simulink model "lab4_task1"  (R2020a)
settings: Solver=FixedStepAuto  StartTime=0.0  StopTime=inf  RelTol=1e-3
model workspace (MAT data in the model file):
  SL_ROS_VariableLengthArrays_MaxSizes.CommonInfo.ArrayTruncateAction = 'EmitWarning'
  SL_ROS_VariableLengthArrays_MaxSizes.MsgTypeMap = containers.Map
  SL_ROS_VariableLengthArrays_MaxSizes.MsgTypeMap.serialization.keys = {'sensor_msgs/LaserScan'}
  SL_ROS_VariableLengthArrays_MaxSizes.MsgTypeMap.serialization.values{1}(1).PropertyName = 'Intensities'
  SL_ROS_VariableLengthArrays_MaxSizes.MsgTypeMap.serialization.values{1}(1).DataType = 'single'
  SL_ROS_VariableLengthArrays_MaxSizes.MsgTypeMap.serialization.values{1}(1).MaxLength = 360
  SL_ROS_VariableLengthArrays_MaxSizes.MsgTypeMap.serialization.values{1}(2).PropertyName = 'Ranges'
  SL_ROS_VariableLengthArrays_MaxSizes.MsgTypeMap.serialization.values{1}(2).DataType = 'single'
  SL_ROS_VariableLengthArrays_MaxSizes.MsgTypeMap.serialization.values{1}(2).MaxLength = 360
  SL_ROS_VariableLengthArrays_MaxSizes.MsgTypeMap.serialization.uniformity = 0
  SL_ROS_VariableLengthArrays_MaxSizes.MsgTypeMap.serialization.keyType = 'char'
  SL_ROS_VariableLengthArrays_MaxSizes.MsgTypeMap.serialization.valueType = 'any'
values from neighbouring files (symbols this model uses):
  theta = ang + curr_yaw    [live_repulsion.m]
undefined symbols (not defined in the file or in its folder): angdiff, Angular, Linear, X, Y
libraries: simulink x9, robotlib x4, robotcorelib x1, simulink_extras x1
settings Model: Creator=Sina  LastModifiedBy=Pablo
settings DataIOCC: ReturnWorkspaceOutputs=off
settings OptimizationCC: EnhancedBackFolding=on  PassReuseOutputArgsAs=Individual arguments  ZeroExternalMemoryAtStartup=off  ZeroInternalMemoryAtStartup=off  MaxStackSize=64  OptimizeBlockOrder=speed  DifferentSizesBufferReuse=on  OptimizationCustomize=off  EfficientTunableParamExpr=on
settings DebuggingCC: ParameterTunabilityLossMsg=error  ArithmeticOperatorsInVariantConditions=warning
settings HardwareCC: ProdBitPerPointer=32  ProdBitPerSizeT=32  ProdBitPerPtrDiffT=32  ProdLargestAtomicFloat=None  ProdIntDivRoundTo=Undefined  ProdEndianess=Unspecified  ProdWordSize=32  ProdHWDeviceType=Generic->Unspecified (assume 32-bit Generic)  UseEmbeddedCoderFeatures=off
settings SFSimCC: SimUseLocalCustomCode=off  MATLABDynamicMemAlloc=off  CustomCodeUndefinedFunction=UseInterfaceOnly
settings RTWCC: SystemTargetFile=ert.tlc  HardwareBoard=Robot Operating System (ROS)  TemplateMakefile=ert_default_tmf  RTWUseLocalCustomCode=off  Toolchain=Catkin  TargetLang=C++
settings CodeAppCC: ForceParamTrailComments=on  IgnoreCustomStorageClasses=off  OperatorAnnotations=on  SimulinkDataObjDesc=on  SFDataObjDesc=on  InsertBlockDesc=on
settings ERTTargetCC: SupportNonInlinedSFcns=on

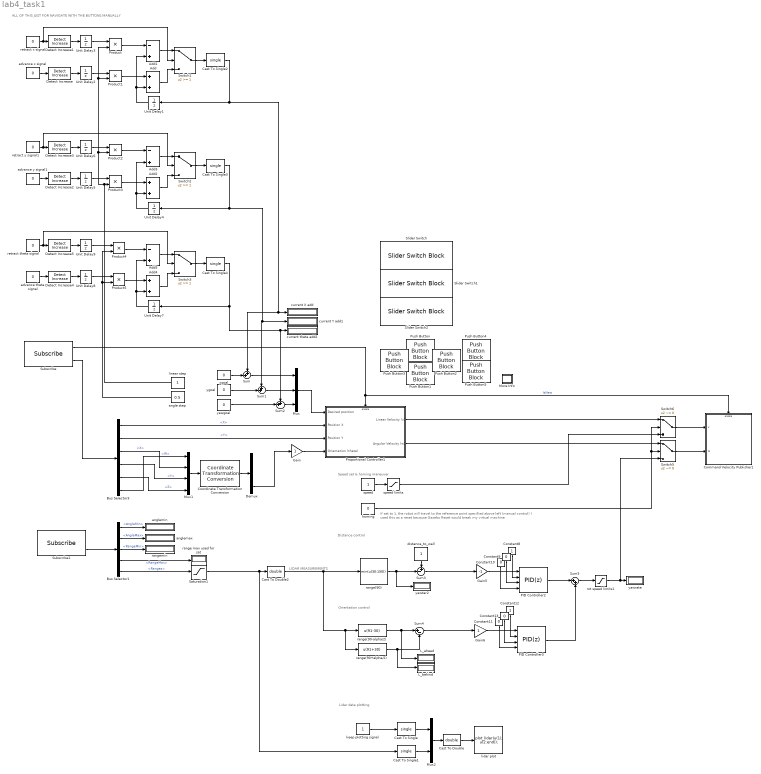
== system lab4_task1 ==
  note: ALL OF THIS JUST FOR NAVIGATE WITH THE BUTTONS MANUALLY
  note: LIDAR MEASUREMENTS
  note: if set to 1, the robot will travel to the reference point specified above left (manual control)
      | I used this as a reset because Gazebo Reset would break my virtual machine
  note: Speed set & homing maneuver
  note: Orientation control
  note: Distance control
  note: Lidar data plotting
  Add : Sum
  Add1 : Sum  Inputs=-+
  Add2 : Sum
  Add3 : Sum  Inputs=-+
  Add4 : Sum
  Add5 : Sum  Inputs=-+
  Bus Selector1 : BusSelector  OutputSignals=AngleMin,AngleMax,RangeMin,RangeMax,Ranges
  Bus Selector3 : BusSelector  OutputSignals=Pose.Pose.Position.X,Pose.Pose.Position.Y,Pose.Pose.Orientation.X,Pose.Pose.Orientation.Y,Pose.Pose.Orientation.Z,Pose.Pose.Orientation.W
  Cast To Double : DataTypeConversion  OutDataTypeStr=double
  Cast To Double2 : DataTypeConversion  OutDataTypeStr=double
  Cast To Single{,1..4} (5 alike) : DataTypeConversion  OutDataTypeStr=single
  Command Velocity Publisher1 : Subsystem
  Constant{9..11,13} (4 alike) : Constant  Value=0
  Constant12 : Constant
  Constant8 : Constant
  Coordinate Transformation Conversion : robotcorelib/Coordinate Transformation Conversion  InputRepresentation=Quaternion  InputEulerSequence=XYZ  ShowTrVecInputPort=on  OutputRepresentation=Euler Angles  OutputEulerSequence=XYZ  ShowTrVecOutputPort=on  SimulateUsing=Interpreted execution
      settings: SourceProductBaseCode=NV,RO,RR
  Demux : Demux  Outputs=3
  Detect Increase{,1..5} (6 alike) : simulink/Logic and Bit Operations/Detect Increase  vinit=0.0  OutDataTypeStr=boolean
  Gain : Gain
  Gain5 : Gain  Gain=-1
  Gain6 : Gain
  L_ahead : Display
  L_behind : Display
  More Info : Subsystem
      settings: OpenFcn=showdemo(bdroot(gcb))
      mask Display: disp('?')
  Mux : Mux  Inputs=3
  Mux1 : Mux
  Mux2 : Mux  Inputs=2
  PID Controller2 : simulink/Continuous/PID Controller  Controller=PID  Form=Parallel  TimeDomain=Discrete-time  UseExternalTs=off  SampleTime=-1  IntegratorMethod=Forward Euler  FilterMethod=Forward Euler  ControllerParametersSource=external  P=1  I=1  D=0  UseFilter=off  N=100  TunerSelectOption=Transfer Function Based (PID Tuner App)  InitialConditionSource=internal  InitialConditionForIntegrator=0  InitialConditionForFilter=0  DifferentiatorICPrevScaledInput=0  ExternalReset=none  TrackingMode=off  Kt=1  LimitOutput=off  UpperSaturationLimit=inf  LowerSaturationLimit=-inf  LinearizeAsGain=on  AntiWindupMode=none  Kb=1  POutMin=[]  POutMax=[]  IOutMin=[]  IOutMax=[]  DOutMin=[]  DOutMax=[]  NOutMin=[]  NOutMax=[]  SumOutMin=[]  SumOutMax=[]  SaturationOutMin=[]  SaturationOutMax=[]  PParamMin=[]  PParamMax=[]  IParamMin=[]  IParamMax=[]  DParamMin=[]  DParamMax=[]  NParamMin=[]  NParamMax=[]  KbParamMin=[]  KbParamMax=[]  KtParamMin=[]  KtParamMax=[]  KbOutMin=[]  KbOutMax=[]  KtOutMin=[]  KtOutMax=[]  IntegratorOutMin=[]  IntegratorOutMax=[]  FilterOutMin=[]  FilterOutMax=[]  SumI1OutMin=[]  SumI1OutMax=[]  SumI2OutMin=[]  SumI2OutMax=[]  SumI3OutMin=[]  SumI3OutMax=[]  SumI4OutMin=[]  SumI4OutMax=[]  SumDOutMin=[]  SumDOutMax=[]  DifferentiatorOutMin=[]  DifferentiatorOutMax=[]  FilterDiffOutCoefMin=[]  FilterDiffOutCoefMax=[]  ReciprocalOutMin=[]  ReciprocalOutMax=[]  SumDenOutMin=[]  SumDenOutMax=[]  SumNumOutMin=[]  SumNumOutMax=[]  DivideOutMin=[]  DivideOutMax=[]  UdiffTsProdOutMin=[]  UdiffTsProdOutMax=[]  NTsProdOutMin=[]  NTsProdOutMax=[]  UintegralTsProdOutMin=[]  UintegralTsProdOutMax=[]  UngainTsProdOutMin=[]  UngainTsProdOutMax=[]  IntegratorContinuousStateAttributes=''  IntegratorStateMustResolveToSignalObject=off  IntegratorRTWStateStorageClass=Auto  FilterContinuousStateAttributes=''  FilterStateMustResolveToSignalObject=off  FilterRTWStateStorageClass=Auto  ParallelPVariant=ExternalParameters  IdealPVariant=Disabled  IVariant=ExternalParameters  DVariant=ExternalParameters  IntegratorVariant=Discrete  SatVariant=Disabled  AWVariant=Passthrough  PCopyVariant=Disabled  TRVariant=Disabled  FdbkBlocksVariant=Forward  IdealPFdbkVariant=Disabled  SatFdbkVariant=Disabled  DerivativeFilterVariant=Differentiator  NVariant=Passthrough  NCopyVariant=Disabled_SignalSpec  FilterICVariant=InternalICsDifferentiator  IntegratorICVariant=InternalICs  ExternalResetVariant=Disabled  TRSumVariant=Passthrough  SumFdbkVariant=Disabled  SumVariant=Sum_PID  TsampFilterVariant=InternalTs  TsampNgainVariant=Passthrough  TsampIntegralVariant=Passthrough
  PID Controller3 : simulink/Continuous/PID Controller  Controller=PID  Form=Parallel  TimeDomain=Discrete-time  UseExternalTs=off  SampleTime=-1  IntegratorMethod=Forward Euler  FilterMethod=Forward Euler  ControllerParametersSource=external  P=1  I=1  D=0  UseFilter=off  N=100  TunerSelectOption=Transfer Function Based (PID Tuner App)  InitialConditionSource=internal  InitialConditionForIntegrator=0  InitialConditionForFilter=0  DifferentiatorICPrevScaledInput=0  ExternalReset=none  TrackingMode=off  Kt=1  LimitOutput=off  UpperSaturationLimit=inf  LowerSaturationLimit=-inf  LinearizeAsGain=on  AntiWindupMode=none  Kb=1  POutMin=[]  POutMax=[]  IOutMin=[]  IOutMax=[]  DOutMin=[]  DOutMax=[]  NOutMin=[]  NOutMax=[]  SumOutMin=[]  SumOutMax=[]  SaturationOutMin=[]  SaturationOutMax=[]  PParamMin=[]  PParamMax=[]  IParamMin=[]  IParamMax=[]  DParamMin=[]  DParamMax=[]  NParamMin=[]  NParamMax=[]  KbParamMin=[]  KbParamMax=[]  KtParamMin=[]  KtParamMax=[]  KbOutMin=[]  KbOutMax=[]  KtOutMin=[]  KtOutMax=[]  IntegratorOutMin=[]  IntegratorOutMax=[]  FilterOutMin=[]  FilterOutMax=[]  SumI1OutMin=[]  SumI1OutMax=[]  SumI2OutMin=[]  SumI2OutMax=[]  SumI3OutMin=[]  SumI3OutMax=[]  SumI4OutMin=[]  SumI4OutMax=[]  SumDOutMin=[]  SumDOutMax=[]  DifferentiatorOutMin=[]  DifferentiatorOutMax=[]  FilterDiffOutCoefMin=[]  FilterDiffOutCoefMax=[]  ReciprocalOutMin=[]  ReciprocalOutMax=[]  SumDenOutMin=[]  SumDenOutMax=[]  SumNumOutMin=[]  SumNumOutMax=[]  DivideOutMin=[]  DivideOutMax=[]  UdiffTsProdOutMin=[]  UdiffTsProdOutMax=[]  NTsProdOutMin=[]  NTsProdOutMax=[]  UintegralTsProdOutMin=[]  UintegralTsProdOutMax=[]  UngainTsProdOutMin=[]  UngainTsProdOutMax=[]  IntegratorContinuousStateAttributes=''  IntegratorStateMustResolveToSignalObject=off  IntegratorRTWStateStorageClass=Auto  FilterContinuousStateAttributes=''  FilterStateMustResolveToSignalObject=off  FilterRTWStateStorageClass=Auto  ParallelPVariant=ExternalParameters  IdealPVariant=Disabled  IVariant=ExternalParameters  DVariant=ExternalParameters  IntegratorVariant=Discrete  SatVariant=Disabled  AWVariant=Passthrough  PCopyVariant=Disabled  TRVariant=Disabled  FdbkBlocksVariant=Forward  IdealPFdbkVariant=Disabled  SatFdbkVariant=Disabled  DerivativeFilterVariant=Differentiator  NVariant=Passthrough  NCopyVariant=Disabled_SignalSpec  FilterICVariant=InternalICsDifferentiator  IntegratorICVariant=InternalICs  ExternalResetVariant=Disabled  TRSumVariant=Passthrough  SumFdbkVariant=Disabled  SumVariant=Sum_PID  TsampFilterVariant=InternalTs  TsampNgainVariant=Passthrough  TsampIntegralVariant=Passthrough
  Product{,1..5} (6 alike) : Product
  Proportional Controller1 : Subsystem
  Push Button : PushButtonBlock  ButtonText=X+
  Push Button1 : PushButtonBlock  ButtonText=X-
  Push Button2 : PushButtonBlock  ButtonText=Y+
  Push Button3 : PushButtonBlock  ButtonText=Y-
  Push Button4 : PushButtonBlock  ButtonText=theta+
  Push Button5 : PushButtonBlock  ButtonText=theta-
  Saturation1 : Saturate  UpperLimit=3.6  LowerLimit=-20  LinearizeAsGain=off
  Slider Switch : SliderSwitchBlock
      settings: Values={{'STOP OFF', 'STOP ON'}, [0 1]}
  Slider Switch1 : SliderSwitchBlock
      settings: Values={{'PLOT OFF', 'PLOT ON'}, [0 1]}
  Slider Switch2 : SliderSwitchBlock
      settings: Values={{'YAW OFF', 'YAW ON'}, [0 -1]}
  Subscribe : robotlib/Subscribe  topicSource=Select from ROS network  topic=/odom  messageType=nav_msgs/Odometry  sampleTime=-1  messageQueueLength=51
  Subscribe1 : robotlib/Subscribe  topicSource=Select from ROS network  topic=/scan  messageType=sensor_msgs/LaserScan  sampleTime=-1  messageQueueLength=51
  Sum : Sum  Inputs=++|
  Sum1 : Sum  Inputs=++|
  Sum2 : Sum  Inputs=++|
  Sum3 : Sum  Inputs=+-|
  Sum4 : Sum  Inputs=|+-
  Sum5 : Sum  Inputs=|++
  Switch1 : Switch  Threshold=1
  Switch2 : Switch  Threshold=1
  Switch3 : Switch  Threshold=1
  Switch5 : Switch  Criteria=u2 ~= 0
  Switch6 : Switch  Criteria=u2 ~= 0
  Unit Delay{1..9} (9 alike) : UnitDelay  SampleTime=-1  HasFrameUpgradeWarning=on
  advance theta signal : Constant  Value=0
  advance x signal : Constant  Value=0
  advance y signal1 : Constant  Value=0
  angle step : Constant  Value=0.5
  anglemax : Display
  anglemin : Display
  current X add : Display
  current Y add1 : Display
  current theta add2 : Display
  distance_to_wall : Constant
  homing : Constant  Value=0
  keep plotting signal : Constant
  lidar plot : MATLABFcn  MATLABFcn=plot_lidar(u(1), u(2:end));  OutputDimensions=1  Output1D=off
  linear step : Constant
  range max used for sat : Display
  range(90) : MATLABFcn  MATLABFcn=min(u(30:150))  OutputDimensions=1  Output1D=off
  range(90+alpha/2) : MATLABFcn  MATLABFcn=u(91+30)  OutputDimensions=1  Output1D=off
  range(90-alpha/2) : MATLABFcn  MATLABFcn=u(91-30)  OutputDimensions=1  Output1D=off
  rangemin : Display
  retract theta signal : Constant  Value=0
  retract x signal : Constant  Value=0
  retract y signal1 : Constant  Value=0
  rot speed limits1 : Saturate  LinearizeAsGain=off
  speed : Constant
  speed limits : Saturate  UpperLimit=0.3  LowerLimit=-0.3  LinearizeAsGain=off
  xgoal : Constant  Value=0
  yawgoal : Constant  Value=0
  yawrate : Display
  yawtar2 : Display
  ygoal : Constant  Value=0
  wires:
  Bus Selector3/2 -> Proportional Controller1/3(Position Y)  "<Y>"
  Bus Selector3/1 -> Proportional Controller1/2(Position X)  "<X>"
  Subscribe/1 -> Command Velocity Publisher1/Enable, Proportional Controller1/Enable  "IsNew"
  Bus Selector3/5 -> Mux1/4  "<Z>"
  Bus Selector3/3 -> Mux1/2  "<X>"
  Subscribe/2 -> Bus Selector3/1
  Bus Selector3/4 -> Mux1/3  "<Y>"
  Bus Selector3/6 -> Mux1/1  "<W>"
  Bus Selector1/2 -> anglemax/1  "<AngleMax>"
  Bus Selector1/5 -> Saturation1/1  "<Ranges>"
  Subscribe1/2 -> Bus Selector1/1
  Bus Selector1/1 -> anglemin/1  "<AngleMin>"
  Mux1/1 -> Coordinate Transformation Conversion/1
  Gain/1 -> Proportional Controller1/4(Orientation (theta))
  Mux/1 -> Proportional Controller1/1(Desired position)
  Coordinate Transformation Conversion/1 -> Demux/1
  Demux/3 -> Gain/1
  Bus Selector1/3 -> rangemin/1  "<RangeMin>"
  Bus Selector1/4 -> range max used for sat/1  "<RangeMax>"
  advance x signal/1 -> Detect Increase/1
  Add/1 -> Switch1/3
  Unit Delay1/1 -> Add/2, Add1/2
  retract x signal/1 -> Switch1/2, Detect Increase1/1
  Add1/1 -> Switch1/1
  Detect Increase/1 -> Unit Delay2/1
  Detect Increase1/1 -> Unit Delay3/1
  Switch1/1 -> Cast To Single2/1
  Cast To Single2/1 -> current X add/1, Sum/1, Unit Delay1/1
  Unit Delay3/1 -> Product/1
  Product/1 -> Add1/1
  Unit Delay2/1 -> Product1/1
  Product1/1 -> Add/1
  Detect Increase2/1 -> Unit Delay5/1
  linear step/1 -> Product/2, Product1/2, Product2/2, Product3/2
  Product2/1 -> Add3/1
  Unit Delay6/1 -> Product2/1
  Switch2/1 -> Cast To Single3/1
  Add3/1 -> Switch2/1
  Unit Delay4/1 -> Add2/2, Add3/2
  Add2/1 -> Switch2/3
  Cast To Single3/1 -> current Y add1/1, Sum1/1, Unit Delay4/1
  Detect Increase3/1 -> Unit Delay6/1
  Unit Delay5/1 -> Product3/1
  retract y signal1/1 -> Switch2/2, Detect Increase3/1
  Product3/1 -> Add2/1
  advance y signal1/1 -> Detect Increase2/1
  Unit Delay7/1 -> Add4/2, Add5/2
  advance theta signal/1 -> Detect Increase4/1
  Product5/1 -> Add4/1
  retract theta signal/1 -> Switch3/2, Detect Increase5/1
  Unit Delay8/1 -> Product5/1
  Cast To Single4/1 -> Sum2/1, current theta add2/1, Unit Delay7/1
  Add4/1 -> Switch3/3
  Add5/1 -> Switch3/1
  Product4/1 -> Add5/1
  Unit Delay9/1 -> Product4/1
  Detect Increase4/1 -> Unit Delay8/1
  Detect Increase5/1 -> Unit Delay9/1
  angle step/1 -> Product4/2, Product5/2
  Switch3/1 -> Cast To Single4/1
  xgoal/1 -> Sum/2
  Sum/1 -> Mux/1
  ygoal/1 -> Sum1/2
  Sum1/1 -> Mux/2
  Sum2/1 -> Mux/3
  speed/1 -> speed limits/1
  yawgoal/1 -> Sum2/2
  speed limits/1 -> Switch6/3
  Switch6/1 -> Command Velocity Publisher1/1(v)
  Switch5/1 -> Command Velocity Publisher1/2(w)
  rot speed limits1/1 -> yawrate/1, Switch5/3
  Proportional Controller1/1(Linear Velocity (v)) -> Switch6/1
  Proportional Controller1/2(Angular Velocity (w)) -> Switch5/1
  homing/1 -> Switch6/2, Switch5/2
  range(90)/1 -> yawtar2/1, Sum3/2
  distance_to_wall/1 -> Sum3/1
  Sum3/1 -> Gain5/1
  Constant9/1 -> PID Controller2/3
  Constant8/1 -> PID Controller2/2
  Constant10/1 -> PID Controller2/4
  PID Controller2/1 -> Sum5/1
  Gain5/1 -> PID Controller2/1
  Sum5/1 -> rot speed limits1/1
  Cast To Double2/1 -> range(90-alpha/2)/1, range(90+alpha/2)/1, range(90)/1
  range(90+alpha/2)/1 -> Sum4/2, L_behind/1
  range(90-alpha/2)/1 -> L_ahead/1, Sum4/1
  Sum4/1 -> Gain6/1
  PID Controller3/1 -> Sum5/2
  Constant11/1 -> PID Controller3/4
  Constant12/1 -> PID Controller3/2
  Constant13/1 -> PID Controller3/3
  Gain6/1 -> PID Controller3/1
  Saturation1/1 -> Cast To Double2/1, Cast To Single1/1
  Cast To Double/1 -> lidar plot/1
  Cast To Single/1 -> Mux2/1
  keep plotting signal/1 -> Cast To Single/1
  Cast To Single1/1 -> Mux2/2
  Mux2/1 -> Cast To Double/1

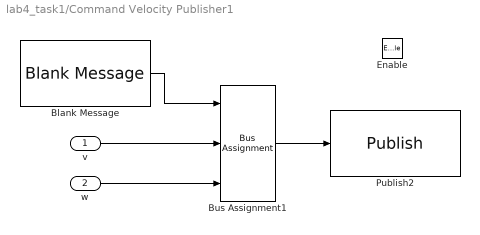
== system lab4_task1/Command Velocity Publisher1 ==
  v : Inport
  w : Inport  Port=2
  Enable : EnablePort
  Blank Message : robotlib/Blank Message  messageClass=Message  entityType=geometry_msgs/Twist  messageType=geometry_msgs/Twist  SampleTime=inf
  Bus Assignment1 : BusAssignment  DialogController=Simulink.DDGSource_BusAssignment  AssignedSignals=Linear.X,Angular.Z
  Publish2 : robotlib/Publish  topicSource=Select from ROS network  topic=/cmd_vel  messageType=geometry_msgs/Twist  messageQueueLength=105
  wires:
  Bus Assignment1/1 -> Publish2/1
  Blank Message/1 -> Bus Assignment1/1
  v/1 -> Bus Assignment1/2
  w/1 -> Bus Assignment1/3

== system lab4_task1/More Info ==

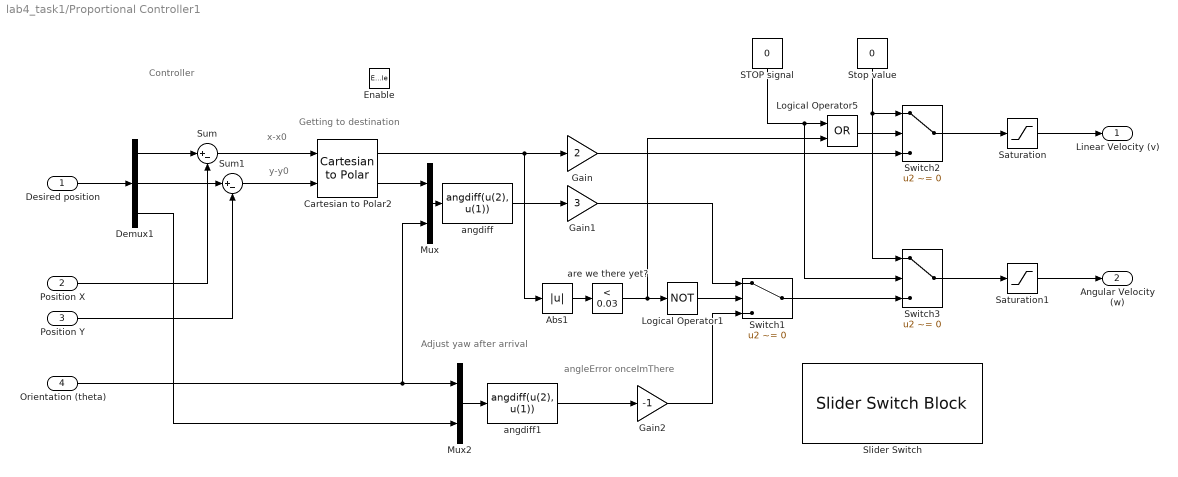
== system lab4_task1/Proportional Controller1 ==
  note: Adjust yaw after arrival
  note: angleError
      | onceImThere
  note: x-x0
  note: y-y0
  note: Controller
  note: Getting to destination
  Desired position : Inport
  Position X : Inport  Port=2
  Position Y : Inport  Port=3
  Orientation (theta) : Inport  Port=4
  Enable : EnablePort
  Abs1 : Abs
  Cartesian to Polar2 : simulink_extras/Transformations/Cartesian to Polar
  Demux1 : Demux  Outputs=3
  Gain : Gain  Gain=2
  Gain1 : Gain  Gain=3
  Gain2 : Gain  Gain=-1
  Logical Operator1 : Logic  Operator=NOT  AllPortsSameDT=off  OutDataTypeStr=boolean
  Logical Operator5 : Logic  Operator=OR  AllPortsSameDT=off  OutDataTypeStr=boolean
  Mux : Mux  Inputs=2
  Mux2 : Mux  Inputs=2
  "STOP signal " : Constant  Value=0
  Saturation : Saturate  UpperLimit=0.3  LowerLimit=-0.3  LinearizeAsGain=off
  Saturation1 : Saturate  UpperLimit=999  LowerLimit=-999  LinearizeAsGain=off
  Slider Switch : SliderSwitchBlock
      settings: Values={{'STOP OFF', 'STOP ON'}, [0 1]}
  Stop value : Constant  Value=0
  Sum : Sum  Inputs=|+-
  Sum1 : Sum  Inputs=|+-
  Switch1 : Switch  Criteria=u2 ~= 0
  Switch2 : Switch  Criteria=u2 ~= 0
  Switch3 : Switch  Criteria=u2 ~= 0
  angdiff : MATLABFcn  MATLABFcn=angdiff(u(2), u(1))  OutputDimensions=1  Output1D=off
  angdiff1 : MATLABFcn  MATLABFcn=angdiff(u(2), u(1))  OutputDimensions=1  Output1D=off
  are we there yet? : simulink/Logic and Bit Operations/Compare To Constant  relop=<  const=0.03  OutDataTypeStr=boolean
  Linear Velocity (v) : Outport  VectorParamsAs1DForOutWhenUnconnected=off
  Angular Velocity (w) : Outport  Port=2  VectorParamsAs1DForOutWhenUnconnected=off
  wires:
  Stop value/1 -> Switch2/1, Switch3/1
  "STOP signal "/1 -> Switch3/2, Logical Operator5/1
  Demux1/1 -> Sum/1
  Demux1/2 -> Sum1/1
  Position Y/1 -> Sum1/2
  Position X/1 -> Sum/2
  Sum/1 -> Cartesian to Polar2/1
  Sum1/1 -> Cartesian to Polar2/2
  Cartesian to Polar2/1 -> Gain/1, Abs1/1
  angdiff/1 -> Gain1/1
  Orientation (theta)/1 -> Mux/2, Mux2/1
  Gain/1 -> Switch2/3
  Mux/1 -> angdiff/1
  Saturation/1 -> Linear Velocity (v)/1
  Switch2/1 -> Saturation/1
  Switch3/1 -> Saturation1/1
  Saturation1/1 -> Angular Velocity (w)/1
  Cartesian to Polar2/2 -> Mux/1
  Desired position/1 -> Demux1/1
  Abs1/1 -> are we there yet?/1
  angdiff1/1 -> Gain2/1
  Mux2/1 -> angdiff1/1
  Demux1/3 -> Mux2/2
  Gain2/1 -> Switch1/3
  Gain1/1 -> Switch1/1
  Switch1/1 -> Switch3/3
  are we there yet?/1 -> Logical Operator1/1, Logical Operator5/2
  Logical Operator1/1 -> Switch1/2
  Logical Operator5/1 -> Switch2/2
